simulink model "EulerAngleController"  (R2022a)
settings: Solver=VariableStepAuto  StartTime=0.0  StopTime=10.0  RelTol=1e-3
values from neighbouring files (symbols this model uses):
  M0inv = inv(M0)    [EulerAngleController.m]
settings Model: Creator=Bruger  LastModifiedBy=Bruger

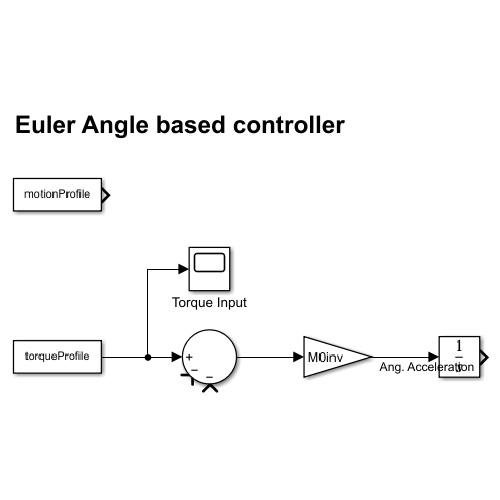
[thumbnail: Simulink's stored preview of the top-level diagram]
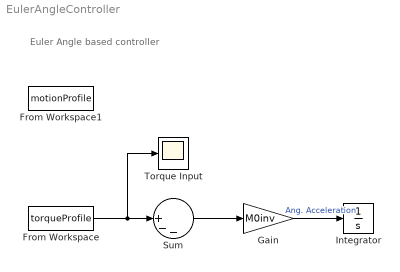
== system EulerAngleController ==
  note: Euler Angle based controller
  From Workspace : FromWorkspace  VariableName=torqueProfile
  From Workspace1 : FromWorkspace  VariableName=motionProfile
  Gain : Gain  Gain=M0inv
  Integrator : Integrator
  Sum : Sum  Inputs=||+--
  Torque Input : Scope
  wires:
  Gain/1 -> Integrator/1  "Ang. Acceleration"
  Sum/1 -> Gain/1
  From Workspace/1 -> Sum/1, Torque Input/1
